simulink model "ROV_Simulator"  (R2023b)
settings: Solver=ode45  StartTime=0.0  StopTime=100  FixedStep=0.0001  MaxStep=0.0001  RelTol=1e-3
InitFcn:
  | init_params
  | 
  | vehicle_parameters_vita1_simu2vita
model workspace (MAT data in the model file):
  PID_params = [219.545279942 3.70519601588 93.8828385991 194.811835155 6.72701520051 121.59112254 154.922739587 1.92908191949 101.939011964 1.23491492885 1.15087256702 0.897835335235 ... (18 elements, 1x18)]
  PID_pitch = [0 0 0]
  PID_roll = [0 0 0]
  PID_x = [0 0 0]
  PID_y = [0 0 0]
  PID_yaw = [0.04 0 0.18]
  PID_z = [0 0 0]
values from neighbouring files (symbols this model uses):
  actuators_tconst = ones(qty_actuators, 1)*0.1754    [vehicle_parameters_vita1_simu2vita.m]
  Dlf = -[X_u;         Y_v;         Z_w;         K_p;         M_q;         N_r]    [vehicle_parameters_vita1_simu2vita.m]
  Dqf = -[X_u_u;         Y_v_v;         Z_w_w;         K_p_p;         M_q_q;         N_r_r]    [vehicle_parameters_vita1_simu2vita.m]
  I_b = diag([I_x; I_y; I_z])    [vehicle_parameters_vita1_simu2vita.m]
  init_vehicle_linear_vel = [0 0 0]'    [init_params.m]
  init_vehicle_position = [0 0 0]'    [init_params.m]
  last_waypoint_thresh = Parameters.reference.path.last_waypoint_thresh    [init_params.m]
  m = 25    [vehicle_parameters_vita1_simu2vita.m]
  Ma = -diag([X_u_dot; Y_v_dot; Z_w_dot; K_p_dot; M_q_dot; N_r_dot])    [vehicle_parameters_vita1_simu2vita.m]
  nlinear_sf = 400    [init_params.m]
  path_ref_mask = Parameters.reference.path.reference_mask    [init_params.m]
  pos_sample_freq = 4    [init_params.m]
  qty_actuators = 8    [vehicle_parameters_vita1_simu2vita.m]
  r_b = [0; 0; -0.08]    [vehicle_parameters_vita1_simu2vita.m]
  r_g = [0; 0; 0.02]    [vehicle_parameters_vita1_simu2vita.m]
  ref_switch = 1    [init_params.m]
  ref_waypoints = Parameters.reference.path.waypoints    [init_params.m]
  rho = 1028    [vehicle_parameters_vita1_simu2vita.m]
  step_signal = Parameters.reference.stage_step_signal    [init_params.m]
  thrust_inferior = ones(qty_actuators, 1)*(-39.91)    [vehicle_parameters_vita1_simu2vita.m]
  thrust_sup = ones(qty_actuators, 1)*51.48    [vehicle_parameters_vita1_simu2vita.m]
  thruster_effectiveness_matrix = thruster_effectiveness_matrix *                               thruster_effectiveness    [vehicle_parameters_vita1_simu2vita.m]
  vol = 0.02432    [vehicle_parameters_vita1_simu2vita.m]
  waypoint_thresh = Parameters.reference.path.waypoint_thresh    [init_params.m]
libraries: slpidlib x6, sharedutil x3, aerolibutil x3, sharedtransform x2, aerolibconvert2 x1, dspswit3 x1
(part 2 of 2)

== matlab function ROV_Simulator/Simu2VITA/Dynamics Module/Kinetics/calculateHydronynamicCoriollisCentripetalMatrix ==
  data: Ca output; nu_r input; m_Ma parameter
function Ca = calculateHydronynamicCoriollisCentripetalMatrix(nu_r, m_Ma)

    [velRow, velCols] = size(nu_r);

    if(velRow == 1 || velCols ~= 1)

        ME = MException('MyComponent:incompatiblePosition', ...
                'Position vector does not match a column vector!');

        throw(ME);

    else

        v = m_Ma*nu_r;
        
        Smtrx_v1 = [0 -v(3) v(2); ... 
                    v(3) 0 -v(1); ... 
                    -v(2) v(1) 0];

        Smtrx_v2 = [0 -v(6) v(5); ... 
                    v(6) 0 -v(4); ... 
                    -v(5) v(4) 0];

        Ca = [zeros(3,3) -Smtrx_v1; ...
              -Smtrx_v1  -Smtrx_v2]; 


    end

end

== matlab function ROV_Simulator/Simu2VITA/Dynamics Module/Kinetics/calculateResultantVelBody ==
  data: nu input; nu_r output; nu_current_dot output; nu_current input
function [nu_r, nu_current_dot] = calculateResultantVelBody(nu, nu_current)
    
   nu_r = nu - [nu_current' 0 0 0]';

   nu_current_dot = [[[0 -nu(6) nu(5); ... 
                       nu(6) 0 -nu(3); ...
                       -nu(5) nu(3) 0]*nu_current]' 0 0 0]';
   
   

end

== matlab function ROV_Simulator/Simu2VITA/Dynamics Module/Kinetics/force_acc ==
  data: C input; Ca input; D input; g input; m_Ma parameter; nu_r input; nu_current_dot input; nu_dot output; nu input; forces output; forces_on_body_components output; tau input; m_M parameter; forces_on_body output
function [nu_dot, forces, forces_on_body_components, forces_on_body] = force_acc(C, Ca, D, g, m_Ma, nu_r, nu_current_dot, nu, tau, m_M)
    
    forces_on_body_components = [m_Ma*nu_current_dot; ...
                                   C*nu; ...
                                 Ca*nu_r; ...
                                 D*nu_r; ...
                                 g];
    forces_on_body = m_Ma*nu_current_dot - C*nu - Ca*nu_r - D*nu_r -  g;
    forces = (tau + forces_on_body);
    nu_dot = (m_M + m_Ma)\forces;
    
end

== matlab function ROV_Simulator/Simu2VITA/Actuator Module/ref_sim_time ==
  data: sim_time input; ref_sim_time output; i_initial_time input; o_initial_time output
function [ref_sim_time, o_initial_time] = ref_sim_time(sim_time, i_initial_time)

        if(i_initial_time == -1)
            i_initial_time = sim_time;
        end

        ref_sim_time = sim_time - i_initial_time;
        o_initial_time =  i_initial_time;
           
end

== matlab function ROV_Simulator/Simu2VITA/Allocation Module/Allocation ==
  data: u_limited input; tau output; thruster_allocation_matrix input
function tau = vehicle_allocation_function(u_limited, thruster_allocation_matrix)

 tau = thruster_allocation_matrix*u_limited;

end

== matlab function ROV_Simulator/Control System/nan-avoider ==
  data: input input; output output size=6
function output = nan_avoider(input)

    output = input;

    for i=1:1:size(input,1)
      
       if (isnan(input(i)))
        output(i) = 0;
       end
       
    end

end

== matlab function ROV_Simulator/Simu2VITA/Actuator Module/first_order_model_actuator ==
  data: u_a output; u_input input; sim_time input; init_actuator_time input
function u_a  = channel_selector(u_input, sim_time, init_actuator_time)

        u_a = u_input.*(sim_time > init_actuator_time);
           
end

== matlab function ROV_Simulator/Simu2VITA/Dynamics Module/Kinetics/calculateDampingMatrix 1 ==
  data: g output; eta input; m_W parameter; m_B parameter; m_r_g parameter; m_r_b parameter
function g = calculateHydrostaticForcesCalculation(eta, m_W, m_B, m_r_g, m_r_b)
            
   coder.extrinsic('MException')
    
    ori = eta(4:7);
    
    g = zeros(6,1);
    
    [Mori, Nori] = size(ori);
    
    if(Mori == 3 && Nori == 1)
        
    elseif(Mori == 4 && Nori == 1)

        q = [eta(4); -eta(5:end)]/norm(eta(4:end));

        S = [0 -q(4) q(3); ...
             q(4) 0 -q(2); ...
            -q(3) q(2) 0;];
        
        r = [0;0;m_W];
        weight_wrt_body = (q(1) - norm(q(2:4)))*r + 2*q(2:4)*(q(2:4)'*r) + 2*q(1)*S*r;
        
        r = [0;0;m_B];
        bouyancy_wrt_body = (q(1) - norm(q(2:4)))*r + 2*q(2:4)*(q(2:4)'*r) + 2*q(1)*S*r;
        
        g(1:3) = -(weight_wrt_body + bouyancy_wrt_body);
        g(4:6) = -(cross(m_r_g, weight_wrt_body) + cross(m_r_b, bouyancy_wrt_body));
        

    end

end

== matlab function ROV_Simulator/Reference Manager/Path Generator/nan-avoider ==
  data: input input; output output size=6
function output = nan_avoider(input)

    output = input;

    for i=1:1:size(input,1)
      
       if (isnan(input(i)))
        output(i) = 0;
       end
       
    end

end

== matlab function ROV_Simulator/Reference Manager/Path Generator/Waypoint Distance  ==
  data: reference input; near_waypoint output; measurement input; error output; waypoint_thresh parameter; last_wpt_check input; last_waypoint_thresh parameter; end_path output; path_ref_mask parameter
function [near_waypoint, error, end_path]= wayp_distance(reference, ...
                                    measurement, waypoint_thresh,  ...
                                    last_wpt_check, last_waypoint_thresh, ...
                                    path_ref_mask)
% WAYP_DISTANCE Determine whether the ROV is getting closer to the next
%               waypoint in the path. Produces a distinct signal when the
%               waypoint is the end of the path.
%
%   Parameters:
%   -----------
%   reference : [Input] (6 x 1 vector) of reference waypoint in the path.
%   measurement : [Input] (6 x 1 vector) of position and attitude 
%                 measurements of the vehicle.
%   waypoint_thresh : [Param] (scalar) acquisition radius to consider a 
%                     waypoint has been reached.
%   last_wpt_check : [Input] (boolean) if 1, announces that the reference 
%                    waypoint is the last waypoint in the path.
%   last_waypoint_thresh : [Param] (scalar) acquisition radius for the last
%   waypoint.
%   path_ref_mask : [Param] (6 x 1 vector) mask vector that determines 
%                   which reference and measurement variables are of 
%                   interest.
%
%   Return:
%   -------
%   near_waypoint : (boolean) 1 if the measured state of the vehicle is
%                   within the acquisiton radius of the current reference
%                   waypoint. This means the next waypoint in the path
%                   should become the target reference.
%   error : (scalar) reference tracking error.
%   end_path : (boolean) 1 if the vehicle has traversed the full path and
%              is within the acquistion radius of the last waypoint. This 
%              means the path following task has come to an end.

    % Init
    near_waypoint = 0;
    end_path = 0;
    % Masking reference and measurements
    masked_ref = reference.*path_ref_mask;
    masked_meas = measurement.*path_ref_mask;
    % Calculating error as an Euclidean distance
    error = norm(masked_ref - masked_meas);
    % If not last waypoint
    if last_wpt_check == 0
        end_path = 0;  % Have not reached the end of the path yet.
        if error <= waypoint_thresh
            near_waypoint = 1;
        end
    else % If last waypoint
        near_waypoint = 0;  % Do not count again.
        if error <= last_waypoint_thresh
            end_path = 1;  % Have reached the end of the path.
        end
    end
end

== matlab function ROV_Simulator/Rotating Control ==
  data: tau_ctrl input; tau output; rot_matrix input
function tau  = control_rotation(tau_ctrl, rot_matrix)
    % roll = rpy(1); pitch = rpy(2); yaw = rpy(3);
    % cr = cos(roll); cp = cos(pitch); cy = cos(yaw);
    % sr = sin(roll); sp = sin(pitch); sy = sin(yaw);
    
    % Rotation matrix ZYX
    % J1 = [cy*cp, cy*sp*sr - sy*cr, cy*sp*cr + sy*sr;
    %       sy*cp, sy*sp*sr + cy*cr, sy*sp*cr - cy*sr;
    %       -sp  , cp*sr           , cp*cr            ];
    % Rotation matrix XYZ
    % J1 = [cp*cy            , -cp*sy           , sp    ;
    %       sr*sp*cy + cr*sy , -sr*sp*sy + cy*cr, -sr*cp;
    %       -cr*sp*cy + sr*sy, cr*sp*sy + sr*cy , cr*cp ];
    
    J1 = rot_matrix;
    % Only rotate in XYZ
    tau = tau_ctrl;
    tau(1:3) = J1*tau_ctrl(1:3);
    tau = tau(:, 1);
end

== matlab function ROV_Simulator/Reference Manager/Path Generator/My Wpt Selector ==
  data: wpts input; ref output; idx input; no_waypoints parameter; last_wpt output
function [ref, last_wpt] = my_selector(wpts, idx, no_waypoints)
    last_wpt = 0;
    % Check idx
    if idx < 1
        idx = 1;
    end
    ref = wpts(:, idx);
    if idx == no_waypoints
        last_wpt = 1;
    end
end

== matlab function ROV_Simulator/Thruster Allocation/Thruster Allocator ==
  data: tau_ref input; u output; control_allocation_matrix parameter
function u = thruster_allocator_function(tau_ref, control_allocation_matrix)
  
  u = control_allocation_matrix*tau_ref;
  % u = thruster_allocation_matrix'/(thruster_allocation_matrix*thruster_allocation_matrix')*tau_ref;
  
end

== matlab function ROV_Simulator/Simu2VITA/Dynamics Module/Kinematics ==
  data: nu input; eta_dot output; eta input
function eta_dot = vita_robot_kinematics(nu, eta)

    R_b2n = [1-2*(eta(6)^2 + eta(7)^2) 2*(eta(5)*eta(6)-eta(7)*eta(4)) 2*(eta(5)*eta(7)+eta(6)*eta(4)); ...
             2*(eta(5)*eta(6)+eta(7)*eta(4)) 1-2*(eta(5)^2 + eta(7)^2) 2*(eta(6)*eta(7)-eta(5)*eta(4)); ...
             2*(eta(5)*eta(7)-eta(6)*eta(4)) 2*(eta(6)*eta(7)+eta(5)*eta(4)) 1-2*(eta(5)^2 + eta(6)^2)];
         
    T = 0.5*[-eta(5) -eta(6) -eta(7); ... 
              eta(4) -eta(7)  eta(6); ...
              eta(7)  eta(4) -eta(5); ...
             -eta(6)  eta(5)  eta(4);];
      
   q = eta(4:7);
   
   eta_dot = zeros(7,1);
   
   %rate of convergence of the quaternion (Chapter 3 of Fossen 2011)
   gamma = 100;
   
   eta_dot(1:3) = R_b2n*nu(1:3);
   eta_dot(4:7) = T*nu(4:6) + (gamma/2)*(1-q'*q)*q;

end

== matlab function ROV_Simulator/Simu2VITA/Dynamics Module/Kinetics/calculateCoriollisCentripetalForceMatrix ==
  data: nu input; C output; m_m parameter; m_r_g parameter; m_I_b parameter
function C = calculateCoriollisCentripetalForceMatrix(nu, m_m, m_r_g, m_I_b)
            
            v2 = nu(4:6);            
            
            Smtrx_v2 = [0 -v2(3) v2(2); ... 
                       v2(3) 0 -v2(1); ... 
                       -v2(2) v2(1) 0];
            
            I_bv2 = m_I_b*v2;
                  
            Smtrx_I_bv2 = [0 -I_bv2(3) I_bv2(2); ... 
                           I_bv2(3) 0 -I_bv2(1); ... 
                          -I_bv2(2) I_bv2(1) 0];
            
            Smtrx_r_g = [0 -m_r_g(3) m_r_g(2); ... 
                         m_r_g(3) 0 -m_r_g(1); ... 
                         -m_r_g(2) m_r_g(1) 0];
                   
            C11 = m_m*Smtrx_v2;
            C12 = -m_m*Smtrx_v2*Smtrx_r_g;
            C21 = m_m*Smtrx_r_g*Smtrx_v2;
            C22 = -Smtrx_I_bv2;
            
            C = [C11 C12; ...
                 C21 C22];
            
end
